simulink model "outdoorAngleFinder"  (R2015b)
settings: Solver=FixedStepAuto  StartTime=0.0  StopTime=10  RelTol=1e-3
libraries: dspsrcs4 x4, dspvision x4, simulink_extras x1, dspstat3 x1
settings Model: Creator=gkeating  LastModifiedBy=gkeating

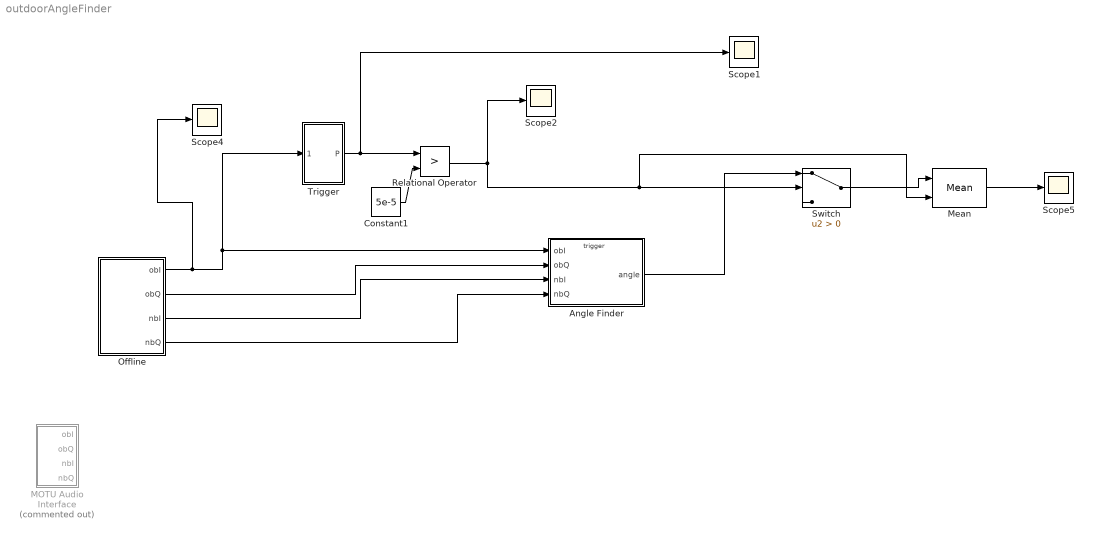
== system outdoorAngleFinder ==
  Angle Finder : Subsystem  TreatAsAtomicUnit=on
  Constant1 : Constant  Value=5e-5  SampleTime=1/192e3
  MOTU Audio Interface : Subsystem  Commented=on
  Mean : dspstat3/Mean  run=on  reset_popup=Either edge  directionMode=Each column  dimension=1  roiEnable=off  roiType=Rectangles  roiPortion=Entire ROI  roiOutput=Individual statistics for each ROI  roiFlag=off  outputDataTypeStr=Inherit: Same as accumulator  outputLastDataTypeStr=Inherit: Same as accumulator  outputMin=[]  outputMax=[]  roundingMode=Floor  overflowMode=off
  Offline : Subsystem
  Relational Operator : RelationalOperator  Operator=>  OutDataTypeStr=boolean
  Scope{1..2,4..5} (4 alike) : Scope
  Switch : Switch  Criteria=u2 > Threshold
  Trigger : Subsystem
  wires:
  Offline/2(obQ) -> Angle Finder/2(obQ)
  Offline/3(nbI) -> Angle Finder/3(nbI)
  Offline/4(nbQ) -> Angle Finder/4(nbQ)
  Trigger/1(P) -> Relational Operator/1, Scope1/1
  Offline/1(obI) -> Scope4/1, Trigger/1(signal), Angle Finder/1(obI)
  Angle Finder/1(angle) -> Switch/1
  Constant1/1 -> Relational Operator/2
  Relational Operator/1 -> Mean/2, Switch/2, Scope2/1
  Switch/1 -> Mean/1
  Mean/1 -> Scope5/1

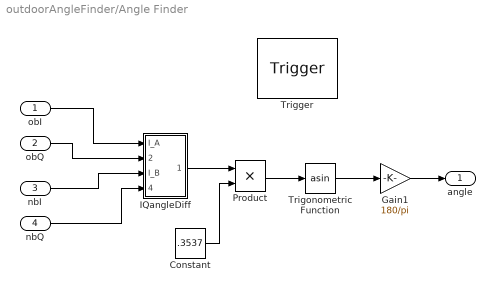
== system outdoorAngleFinder/Angle Finder ==
  obI : Inport
  obQ : Inport  Port=2
  nbI : Inport  Port=3
  nbQ : Inport  Port=4
  Trigger : TriggerPort  TriggerType=either  PortDimensions=1
  Constant : Constant  Value=.3537  SampleTime=-1
  Gain1 : Gain  Gain=180/pi
  IQangleDiff : Subsystem
  Product : Product
  Trigonometric Function : Trigonometry  Operator=asin
  angle : Outport
  wires:
  IQangleDiff/1(A-B) -> Product/1
  Product/1 -> Trigonometric Function/1
  Trigonometric Function/1 -> Gain1/1
  Constant/1 -> Product/2
  Gain1/1 -> angle/1
  obI/1 -> IQangleDiff/1(I_A)
  obQ/1 -> IQangleDiff/2(Q_A)
  nbI/1 -> IQangleDiff/3(I_B)
  nbQ/1 -> IQangleDiff/4(Q_B)

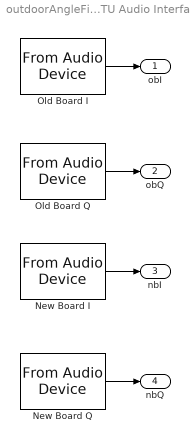
== system outdoorAngleFinder/MOTU Audio Interface ==
  New Board I : dspsrcs4/From Audio Device  deviceName=MOTU Traveler  numChannels=1  sampleRate=192000  deviceDatatype=Determine from output data type  autoBufferSize=on  bufferSize=4096  queueDuration=1.0  frameSize=1  outputDatatype=double  defaultInputChannelMapping=off  inputChannelMapping=7  outputNumOverrunSamples=off  OutputFrames=off
  New Board Q : dspsrcs4/From Audio Device  deviceName=MOTU Traveler  numChannels=1  sampleRate=192000  deviceDatatype=Determine from output data type  autoBufferSize=on  bufferSize=4096  queueDuration=1.0  frameSize=1  outputDatatype=double  defaultInputChannelMapping=off  inputChannelMapping=8  outputNumOverrunSamples=off  OutputFrames=off
  Old Board I : dspsrcs4/From Audio Device  deviceName=MOTU Traveler  numChannels=1  sampleRate=192000  deviceDatatype=Determine from output data type  autoBufferSize=on  bufferSize=4096  queueDuration=1.0  frameSize=1  outputDatatype=double  defaultInputChannelMapping=off  inputChannelMapping=5  outputNumOverrunSamples=off  OutputFrames=off
  Old Board Q : dspsrcs4/From Audio Device  deviceName=MOTU Traveler  numChannels=1  sampleRate=192000  deviceDatatype=Determine from output data type  autoBufferSize=on  bufferSize=4096  queueDuration=1.0  frameSize=1  outputDatatype=double  defaultInputChannelMapping=off  inputChannelMapping=6  outputNumOverrunSamples=off  OutputFrames=off
  obI : Outport
  obQ : Outport  Port=2
  nbI : Outport  Port=3
  nbQ : Outport  Port=4
  wires:
  New Board Q/1 -> nbQ/1
  New Board I/1 -> nbI/1
  Old Board I/1 -> obI/1
  Old Board Q/1 -> obQ/1

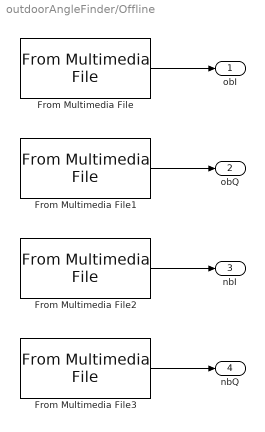
== system outdoorAngleFinder/Offline ==
  From Multimedia File : dspvision/From Multimedia File  inputFilename=/Users/gkeating/Desktop/simtest/obI.wav  loop=on  numPlays=1  outputStreams=Audio only  videoDataType=single  audioDataType=double  inheritSampleTime=on  userDefinedSampleTime=1/30  noAudioOutput=off  isIntensityVideo=off  fourcc=RGB  colorVideoFormat=Separate color signals  outputEOF=off  dataOrg=Column-major  audioFrameSize=1  computeAudioFrameSize=off  outSamplingMode=Sample based
  From Multimedia File1 : dspvision/From Multimedia File  inputFilename=/Users/gkeating/Desktop/simtest/obQ.wav  loop=on  numPlays=1  outputStreams=Audio only  videoDataType=single  audioDataType=double  inheritSampleTime=on  userDefinedSampleTime=1/30  noAudioOutput=off  isIntensityVideo=off  fourcc=RGB  colorVideoFormat=Separate color signals  outputEOF=off  dataOrg=Column-major  audioFrameSize=1  computeAudioFrameSize=off  outSamplingMode=Sample based
  From Multimedia File2 : dspvision/From Multimedia File  inputFilename=/Users/gkeating/Desktop/simtest/nbI.wav  loop=on  numPlays=1  outputStreams=Audio only  videoDataType=single  audioDataType=double  inheritSampleTime=on  userDefinedSampleTime=1/30  noAudioOutput=off  isIntensityVideo=off  fourcc=RGB  colorVideoFormat=Separate color signals  outputEOF=off  dataOrg=Column-major  audioFrameSize=1  computeAudioFrameSize=off  outSamplingMode=Sample based
  From Multimedia File3 : dspvision/From Multimedia File  inputFilename=/Users/gkeating/Desktop/simtest/nbQ.wav  loop=on  numPlays=1  outputStreams=Audio only  videoDataType=single  audioDataType=double  inheritSampleTime=on  userDefinedSampleTime=1/30  noAudioOutput=off  isIntensityVideo=off  fourcc=RGB  colorVideoFormat=Separate color signals  outputEOF=off  dataOrg=Column-major  audioFrameSize=1  computeAudioFrameSize=off  outSamplingMode=Sample based
  obI : Outport
  obQ : Outport  Port=2
  nbI : Outport  Port=3
  nbQ : Outport  Port=4
  wires:
  From Multimedia File3/1 -> nbQ/1
  From Multimedia File2/1 -> nbI/1
  From Multimedia File/1 -> obI/1
  From Multimedia File1/1 -> obQ/1

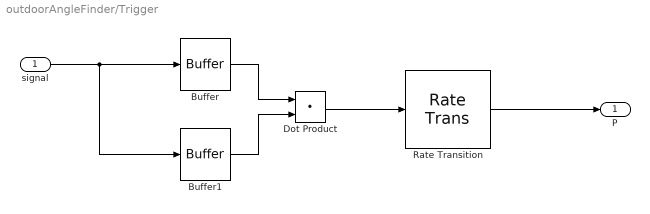
== system outdoorAngleFinder/Trigger ==
  signal : Inport
  Buffer : Buffer  N=30  TreatMby1Signals=One channel  OutputFrames=off
  Buffer1 : Buffer  N=30  TreatMby1Signals=One channel  OutputFrames=off
  Dot Product : DotProduct  InputSameDT=on
  Rate Transition : RateTransition  OutPortSampleTimeMultiple=1/30  OutPortSampleTime=1/192e3
  P : Outport
  wires:
  Buffer/1 -> Dot Product/1
  signal/1 -> Buffer/1, Buffer1/1
  Buffer1/1 -> Dot Product/2
  Dot Product/1 -> Rate Transition/1
  Rate Transition/1 -> P/1

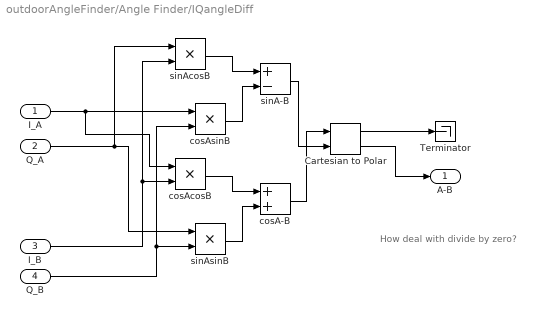
== system outdoorAngleFinder/Angle Finder/IQangleDiff ==
  note: How deal with divide by zero?
  I_A : Inport
  Q_A : Inport  Port=2
  I_B : Inport  Port=3
  Q_B : Inport  Port=4
  Cartesian to Polar : simulink_extras/Transformations/Cartesian to Polar
  Terminator : Terminator
  cosA-B : Sum
  cosAcosB : Product
  cosAsinB : Product
  sinA-B : Sum  Inputs=+-
  sinAcosB : Product
  sinAsinB : Product
  A-B : Outport
  wires:
  I_B/1 -> sinAcosB/2, cosAcosB/2
  sinAcosB/1 -> sinA-B/1
  sinA-B/1 -> Cartesian to Polar/2
  sinAsinB/1 -> cosA-B/2
  Q_A/1 -> sinAsinB/1, sinAcosB/1
  cosA-B/1 -> Cartesian to Polar/1
  I_A/1 -> cosAcosB/1, cosAsinB/1
  Cartesian to Polar/1 -> Terminator/1
  Q_B/1 -> sinAsinB/2, cosAsinB/2
  Cartesian to Polar/2 -> A-B/1
  cosAsinB/1 -> sinA-B/2
  cosAcosB/1 -> cosA-B/1
